simulink model "model"  (R2015b)
settings: Solver=VariableStepAuto  StartTime=0.0  StopTime=5  RelTol=1e-3
StartFcn:
  | global con;
  | con = constants;
settings Model: Creator=petter  LastModifiedBy=petter

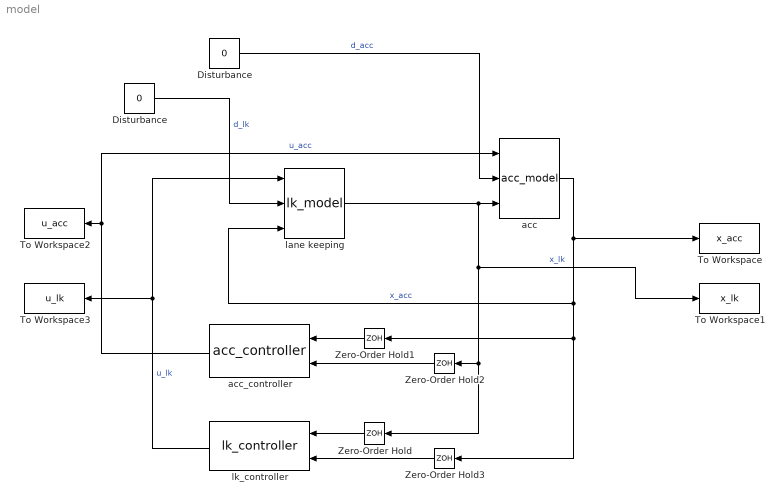
== system model ==
  Disturbance : Constant  Value=0
  "Disturbance " : Constant  Value=0
  To Workspace : ToWorkspace  VariableName=x_acc  SaveFormat=Timeseries  SampleTime=-1
  To Workspace1 : ToWorkspace  VariableName=x_lk  SaveFormat=Timeseries  SampleTime=-1
  To Workspace2 : ToWorkspace  VariableName=u_acc  SaveFormat=Timeseries  SampleTime=-1
  To Workspace3 : ToWorkspace  VariableName=u_lk  SaveFormat=Timeseries  SampleTime=-1
  Zero-Order Hold{,1..3} (4 alike) : ZeroOrderHold  SampleTime=0.01
  acc : M-S-Function  FunctionName=acc_model
  acc_controller : M-S-Function  FunctionName=acc_controller
  "lane keeping " : M-S-Function  FunctionName=lk_model
  lk_controller : M-S-Function  FunctionName=lk_controller
  wires:
  acc/1 -> "lane keeping "/3, Zero-Order Hold1/1, Zero-Order Hold3/1, To Workspace/1  "x_acc"
  "lane keeping "/1 -> Zero-Order Hold/1, Zero-Order Hold2/1, To Workspace1/1, acc/3  "x_lk"
  "Disturbance "/1 -> "lane keeping "/2  "d_lk"
  acc_controller/1 -> To Workspace2/1, acc/1  "u_acc"
  lk_controller/1 -> To Workspace3/1, "lane keeping "/1  "u_lk"
  Disturbance/1 -> acc/2  "d_acc"
  Zero-Order Hold/1 -> lk_controller/1
  Zero-Order Hold3/1 -> lk_controller/2
  Zero-Order Hold1/1 -> acc_controller/1
  Zero-Order Hold2/1 -> acc_controller/2
